simulink model "multiAgents3"  (Simulink 7.0)
settings: Solver=ode23t  StartTime=0.0  StopTime=5  RelTol=1e-3
values from neighbouring files (symbols this model uses):
  A = [Lg1Lfh1 Lg2Lfh1; Lg1Lfh2 Lg2Lfh2]    [example.m]    (also in initMultiAgents.m = kron(eye(6),Ai); linearization.m; makeIncludedAngleMatrix.m = zeros(l,l); unicycle.m)
  A1 = toMatrix(block.InputPort(1).Data)    [assignmentDynamics.m]    (also in initMultiAgents.m = makeIncludedAngleMatrix(zeta))
  A2 = toMatrix(block.InputPort(2).Data)    [assignmentDynamics.m]    (also in initMultiAgents.m = makeIncludedAngleMatrix(tmp))
  B = kron(eye(6),Bi)    [initMultiAgents.m]
  C = kron(eye(6),Ci)    [initMultiAgents.m]
  D = kron(eye(6),Di)    [initMultiAgents.m]
  initZ = [z01, z02, z03, z04, z05, z06].'    [initMultiAgents.m]
  K1 = kron(eye(6),[k11 0;0 k12])    [initMultiAgents.m]
  K2 = kron(eye(6),[k21 0;0 k22])    [initMultiAgents.m]
  Lm = kron(L,eye(2))    [initMultiAgents.m]
  zeta = [0 0 -100 -200 100 -200 -200 -400 0 -400 200 -400].'    [initMultiAgents.m]
libraries: simulink x2
settings Model: Creator=wizest  LastModifiedBy=wizest

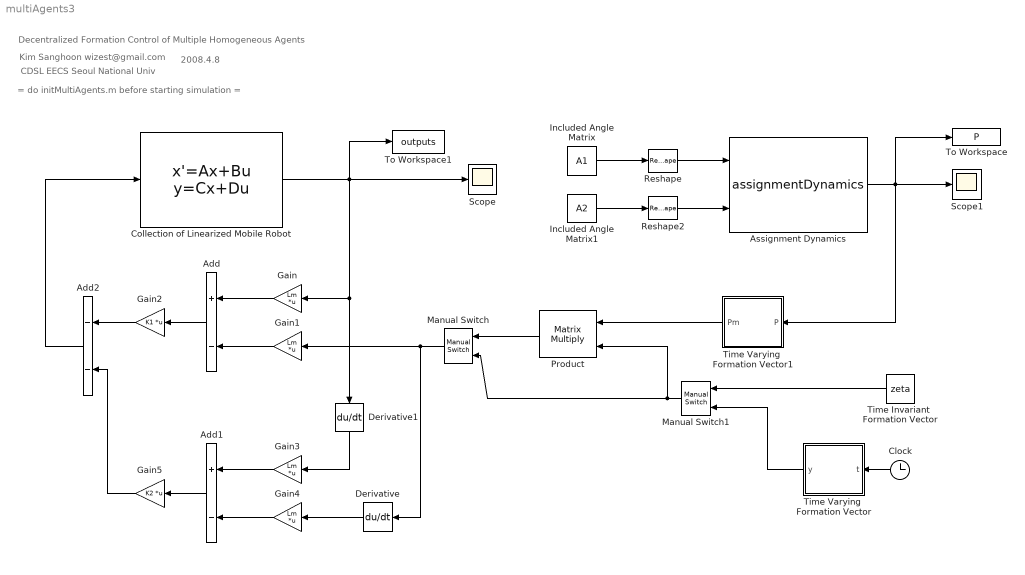
== system multiAgents3 ==
  note: = do initMultiAgents.m before starting simulation =
  note: Kim Sanghoon wizest@gmail.com
  note: 2008.4.8
  note: CDSL EECS Seoul National Univ
  note: Decentralized Formation Control of Multiple Homogeneous Agents
  Add : Sum  Orientation=left  Inputs=+-  OutDataType=sfix(16)  OutScaling=2^-10
  Add1 : Sum  Orientation=left  Inputs=+-  OutDataType=sfix(16)  OutScaling=2^-10
  Add2 : Sum  Orientation=left  Inputs=--  OutDataType=sfix(16)  OutScaling=2^-10
  Assignment Dynamics : M-S-Function  FunctionName=assignmentDynamics
  Clock : Clock
      settings: Decimation=10
  Collection of Linearized Mobile Robot : StateSpace  A=A  B=B  C=C  D=D  X0=initZ
  Derivative : Derivative  Orientation=left
  Derivative1 : Derivative  Orientation=down
  Gain{,1,3..4} (4 alike) : Gain  Orientation=left  Gain=Lm  Multiplication=Matrix(K*u) (u vector)  ParameterDataType=sfix(16)  ParameterScaling=2^0  OutDataType=sfix(16)  OutScaling=2^0
  Gain2 : Gain  Orientation=left  Gain=K1  Multiplication=Matrix(K*u) (u vector)  ParameterDataType=sfix(16)  ParameterScaling=2^0  OutDataType=sfix(16)  OutScaling=2^0
  Gain5 : Gain  Orientation=left  Gain=K2  Multiplication=Matrix(K*u) (u vector)  ParameterDataType=sfix(16)  ParameterScaling=2^0  OutDataType=sfix(16)  OutScaling=2^0
  Included Angle Matrix : Constant  Value=A1  OutDataType=sfix(16)  OutScaling=2^0
  Included Angle Matrix1 : Constant  Value=A2  OutDataType=sfix(16)  OutScaling=2^0
  Manual Switch : simulink/Signal Routing/Manual Switch  Orientation=left  SystemSampleTime=-1  sw=0  action=0  varsize=off
  Manual Switch1 : simulink/Signal Routing/Manual Switch  Orientation=left  SystemSampleTime=-1  sw=0  action=0  varsize=off
  Product : Product  Orientation=left  Multiplication=Matrix(*)  OutDataType=sfix(16)  OutScaling=2^0  RndMeth=Zero
  Reshape : Reshape  OutputDimensionality=Column vector (2-D)
  Reshape2 : Reshape  OutputDimensionality=Column vector (2-D)
  Scope : Scope
      settings: TimeRange=5  YMin=-600  YMax=600
  Scope1 : Scope
      settings: TimeRange=10  YMin=-0.1  YMax=1
  Time Invariant  Formation Vector : Constant  Orientation=left  Value=zeta  OutDataType=sfix(16)  OutScaling=2^0
  Time Varying  Formation Vector : Stateflow chart  Orientation=left
  Time Varying  Formation Vector1 : Stateflow chart  Orientation=left
  To Workspace : ToWorkspace  VariableName=P  SampleTime=-1  SaveFormat=Structure
  To Workspace1 : ToWorkspace  VariableName=outputs  SampleTime=-1  SaveFormat=Structure
  wires:
  Collection of Linearized Mobile Robot/1 -> Gain/1, Derivative1/1, Scope/1, To Workspace1/1
  Gain/1 -> Add/1
  Gain1/1 -> Add/2
  Add/1 -> Gain2/1
  Gain3/1 -> Add1/1
  Gain4/1 -> Add1/2
  Add1/1 -> Gain5/1
  Gain2/1 -> Add2/1
  Gain5/1 -> Add2/2
  Add2/1 -> Collection of Linearized Mobile Robot/1
  Derivative/1 -> Gain4/1
  Derivative1/1 -> Gain3/1
  Clock/1 -> Time Varying  Formation Vector/1(t)
  Manual Switch/1 -> Gain1/1, Derivative/1
  Manual Switch1/1 -> Manual Switch/2, Product/2
  Assignment Dynamics/1 -> Scope1/1, Time Varying  Formation Vector1/1(P), To Workspace/1
  Reshape/1 -> Assignment Dynamics/1
  Included Angle Matrix/1 -> Reshape/1
  Included Angle Matrix1/1 -> Reshape2/1
  Reshape2/1 -> Assignment Dynamics/2
  Product/1 -> Manual Switch/1
  Time Varying  Formation Vector1/1(Pm) -> Product/1
  Time Invariant  Formation Vector/1 -> Manual Switch1/1
  Time Varying  Formation Vector/1(y) -> Manual Switch1/2

== matlab function Time Varying Formation Vector1 ==
  data: P input inherited; Pm output inherited
function Pm = fcn(P)
Pm = kron(toMatrix(P),eye(2));

== matlab function Time Varying Formation Vector ==
  data: t input inherited; y output inherited
function y = fcn(t)
zeta=[  0;                  0;
        -100-50*sin(t);    -200-100*sin(t);
        100+50*sin(t);     -200-100*sin(t);
        -200-100*sin(t);    -400-200*sin(t);
        0;                  -400-200*sin(t);
        200+100*sin(t);     -400-200*sin(t)];
y = zeta;
